simulink library "EoM_6DoF"  (R2021b)
settings: Solver=VariableStepAuto  StartTime=0.0  StopTime=10.0  RelTol=1e-3
undefined symbols (not defined in the file or in its folder): g, p0, phi0, psi0, q0, r0, theta0, u0, v0, w0, X0, Y0, Z0
libraries: EqMpro x12
settings Model: Creator=setup  LastModifiedBy=dmgp1

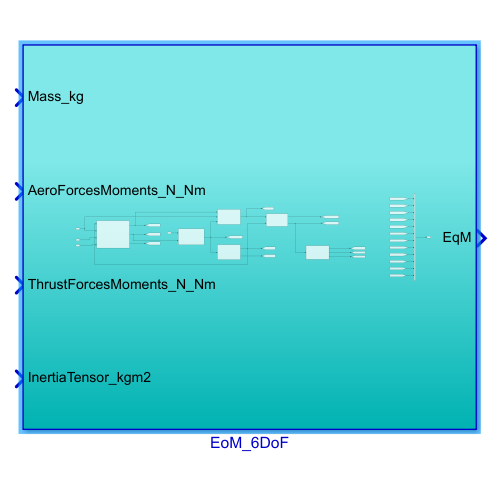
[thumbnail: Simulink's stored preview of the top-level diagram]
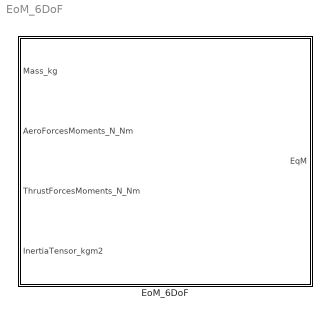
== system EoM_6DoF ==
  EoM_6DoF : Subsystem

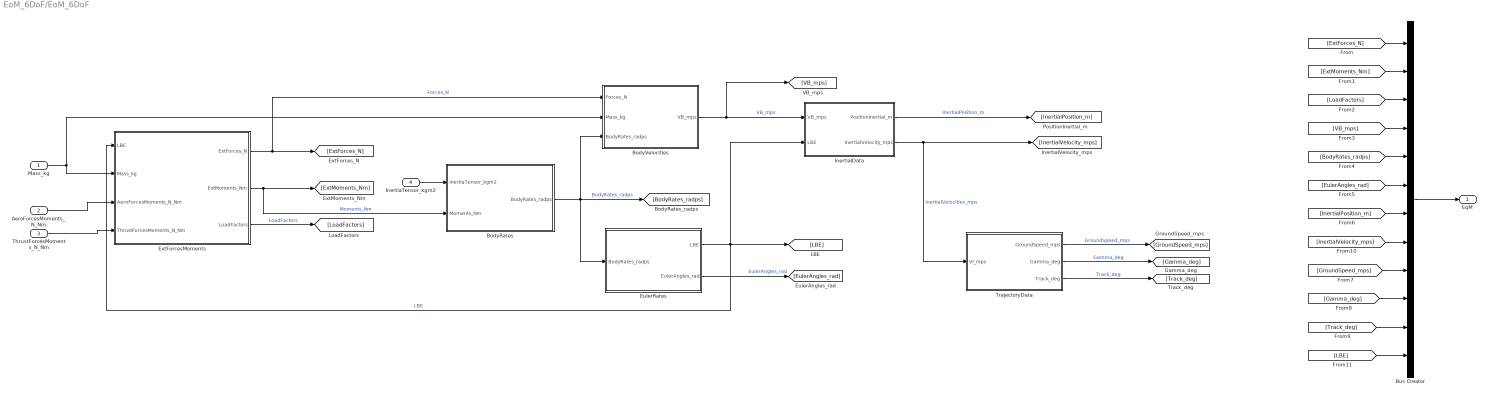
== system EoM_6DoF/EoM_6DoF ==
  Mass_kg : Inport  PortDimensions=[1]
  AeroForcesMoments_N_Nm : Inport  Port=2  PortDimensions=[6]
  ThrustForcesMoments_N_Nm : Inport  Port=3  PortDimensions=[6]
  InertiaTensor_kgm2 : Inport  Port=4
  BodyRates : Subsystem
  BodyVelocities : Subsystem
  Bus Creator : BusCreator  Inputs=12
  EulerRates : Subsystem
  ExtForcesMoments : Subsystem
  InertialData : Subsystem
  TrajectoryData : Subsystem
  EqM : Outport
  wires:
  ExtForcesMoments/3(LoadFactors) -> [LoadFactors]  "LoadFactors"
  BodyVelocities/1(VB_mps) -> [VB_mps], InertialData/1(VB_mps)  "VB_mps"
  [LBE] -> Bus Creator/12
  ThrustForcesMoments_N_Nm/1 -> ExtForcesMoments/4(ThrustForcesMoments_N_Nm)
  [Track_deg] -> Bus Creator/11
  Bus Creator/1 -> EqM/1
  TrajectoryData/3(Track_deg) -> [Track_deg]  "Track_deg"
  AeroForcesMoments_N_Nm/1 -> ExtForcesMoments/3(AeroForcesMoments_N_Nm)
  [ExtForces_N] -> Bus Creator/1
  ExtForcesMoments/1(ExtForces_N) -> BodyVelocities/1(Forces_N), [ExtForces_N]  "Forces_N"
  [Gamma_deg] -> Bus Creator/10
  [LoadFactors] -> Bus Creator/3
  [InertialPosition_m] -> Bus Creator/7
  [VB_mps] -> Bus Creator/4
  BodyRates/1(BodyRates_radps) -> [BodyRates_radps], EulerRates/1(BodyRates_radps), BodyVelocities/3(BodyRates_radps)  "BodyRates_radps"
  Mass_kg/1 -> ExtForcesMoments/2(Mass_kg), BodyVelocities/2(Mass_kg)
  EulerRates/1(LBE) -> ExtForcesMoments/1(LBE), [LBE], InertialData/2(LBE)  "LBE"
  InertialData/1(PositionInertial_m) -> [InertialPosition_m]  "InertialPosition_m"
  ExtForcesMoments/2(ExtMoments_Nm) -> BodyRates/2(Moments_Nm), [ExtMoments_Nm]  "Moments_Nm"
  [GroundSpeed_mps] -> Bus Creator/9
  EulerRates/2(EulerAngles_rad) -> [EulerAngles_rad]  "EulerAngles_rad"
  [InertialVelocity_mps] -> Bus Creator/8
  InertialData/2(InertialVelocity_mps) -> [InertialVelocity_mps], TrajectoryData/1(VI_mps)  "InertialVelocities_mps"
  [ExtMoments_Nm] -> Bus Creator/2
  TrajectoryData/2(Gamma_deg) -> [Gamma_deg]  "Gamma_deg"
  InertiaTensor_kgm2/1 -> BodyRates/1(InertiaTensor_kgm2)
  [EulerAngles_rad] -> Bus Creator/6
  [BodyRates_radps] -> Bus Creator/5
  TrajectoryData/1(GroundSpeed_mps) -> [GroundSpeed_mps]  "GroundSpeed_mps"

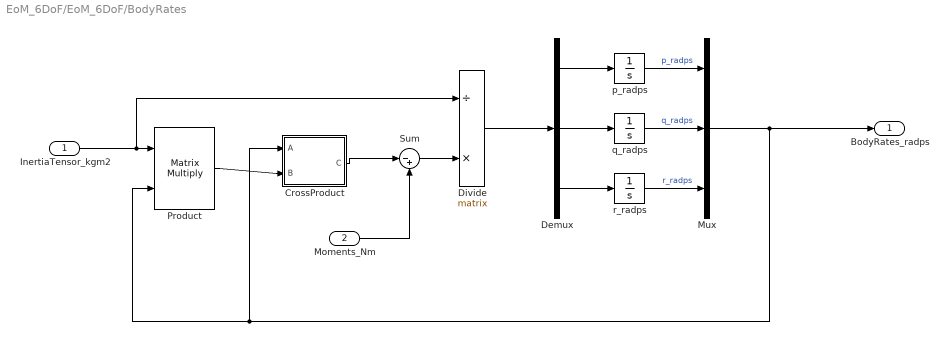
== system EoM_6DoF/EoM_6DoF/BodyRates ==
  InertiaTensor_kgm2 : Inport
  Moments_Nm : Inport  Port=2  PortDimensions=[3]
  CrossProduct : Subsystem
  Demux : Demux  Outputs=3
  Divide : Product  Inputs=/*  Multiplication=Matrix(*)
  Mux : Mux  Inputs=3
  Product : Product  Multiplication=Matrix(*)
  Sum : Sum  Inputs=|-+
  p_radps : Integrator  InitialCondition=p0  ContinuousStateAttributes='p_radps'
  q_radps : Integrator  InitialCondition=q0  ContinuousStateAttributes='q_radps'
  r_radps : Integrator  InitialCondition=r0  ContinuousStateAttributes='r_radps'
  BodyRates_radps : Outport  PortDimensions=[3]
  wires:
  Demux/3 -> r_radps/1
  InertiaTensor_kgm2/1 -> Divide/1, Product/1
  Mux/1 -> BodyRates_radps/1, Product/2, CrossProduct/1(A)
  Product/1 -> CrossProduct/2(B)
  Moments_Nm/1 -> Sum/2
  r_radps/1 -> Mux/3  "r_radps"
  CrossProduct/1(C) -> Sum/1
  Sum/1 -> Divide/2
  q_radps/1 -> Mux/2  "q_radps"
  Demux/1 -> p_radps/1
  p_radps/1 -> Mux/1  "p_radps"
  Demux/2 -> q_radps/1
  Divide/1 -> Demux/1

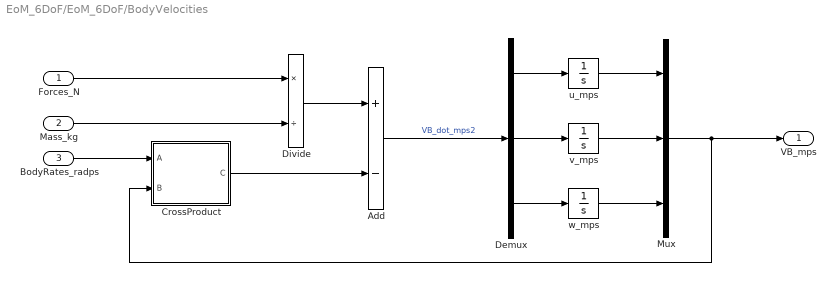
== system EoM_6DoF/EoM_6DoF/BodyVelocities ==
  Forces_N : Inport  PortDimensions=[3]
  Mass_kg : Inport  Port=2  PortDimensions=[1]
  BodyRates_radps : Inport  Port=3  PortDimensions=[3]
  Add : Sum  Inputs=+-
  CrossProduct : Subsystem
  Demux : Demux  Outputs=3
  Divide : Product  Inputs=*/
  Mux : Mux  Inputs=3
  u_mps : Integrator  InitialCondition=u0  ContinuousStateAttributes='u_mps'
  v_mps : Integrator  InitialCondition=v0  ContinuousStateAttributes='v_mps'
  w_mps : Integrator  InitialCondition=w0  ContinuousStateAttributes='w_mps'
  VB_mps : Outport  PortDimensions=[3]
  wires:
  Mux/1 -> VB_mps/1, CrossProduct/2(B)
  Forces_N/1 -> Divide/1
  u_mps/1 -> Mux/1
  Mass_kg/1 -> Divide/2
  Add/1 -> Demux/1  "VB_dot_mps2"
  Divide/1 -> Add/1
  w_mps/1 -> Mux/3
  Demux/1 -> u_mps/1
  CrossProduct/1(C) -> Add/2
  Demux/2 -> v_mps/1
  Demux/3 -> w_mps/1
  v_mps/1 -> Mux/2
  BodyRates_radps/1 -> CrossProduct/1(A)

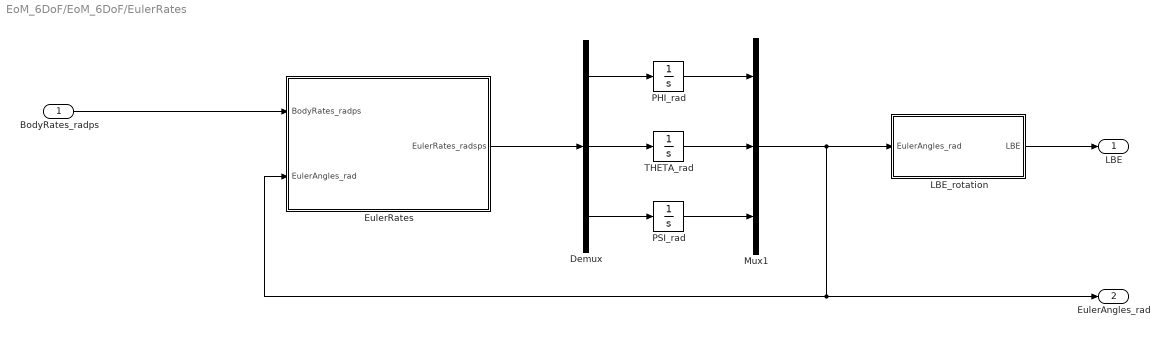
== system EoM_6DoF/EoM_6DoF/EulerRates ==
  BodyRates_radps : Inport  PortDimensions=[3]
  Demux : Demux  Outputs=3
  EulerRates : Subsystem
  LBE_rotation : Subsystem
  Mux1 : Mux  Inputs=3
  PHI_rad : Integrator  InitialCondition=phi0  ContinuousStateAttributes='PHI_rad'
  PSI_rad : Integrator  InitialCondition=psi0  ContinuousStateAttributes='PSI_rad'
  THETA_rad : Integrator  InitialCondition=theta0  ContinuousStateAttributes='THETA_rad'
  LBE : Outport
  EulerAngles_rad : Outport  Port=2
  wires:
  Mux1/1 -> EulerAngles_rad/1, EulerRates/2(EulerAngles_rad), LBE_rotation/1(EulerAngles_rad)
  LBE_rotation/1(LBE) -> LBE/1
  PHI_rad/1 -> Mux1/1
  EulerRates/1(EulerRates_radsps) -> Demux/1
  THETA_rad/1 -> Mux1/2
  PSI_rad/1 -> Mux1/3
  Demux/2 -> THETA_rad/1
  Demux/3 -> PSI_rad/1
  Demux/1 -> PHI_rad/1
  BodyRates_radps/1 -> EulerRates/1(BodyRates_radps)

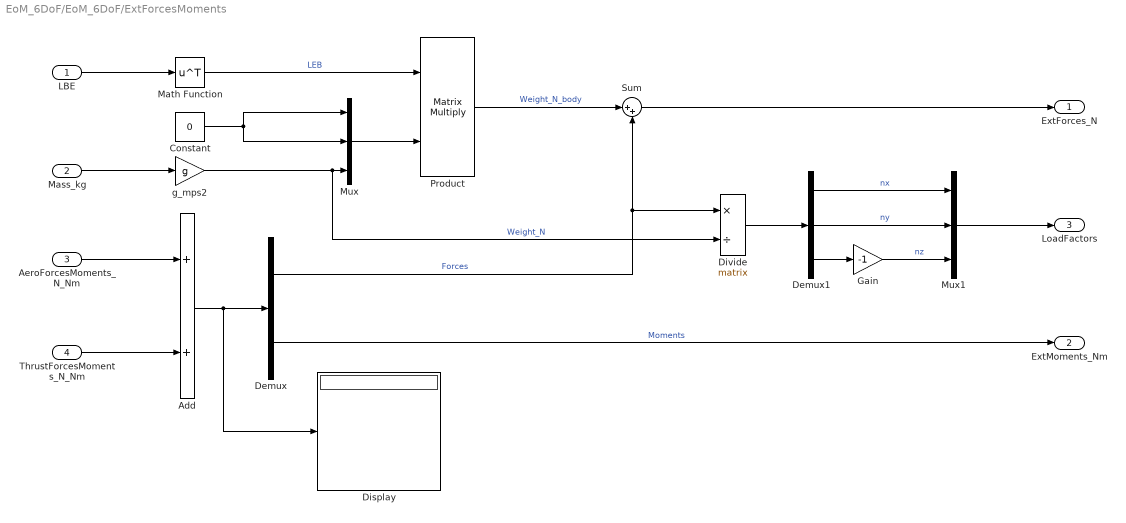
== system EoM_6DoF/EoM_6DoF/ExtForcesMoments ==
  LBE : Inport
  Mass_kg : Inport  Port=2  PortDimensions=[1]
  AeroForcesMoments_N_Nm : Inport  Port=3  PortDimensions=[6]
  ThrustForcesMoments_N_Nm : Inport  Port=4  PortDimensions=[6]
  Add : Sum
  Constant : Constant  Value=0
  Demux : Demux  Outputs=2
  Demux1 : Demux  Outputs=3
  Display : Display
  Divide : Product  Inputs=*/  Multiplication=Matrix(*)
  Gain : Gain  Gain=-1
  Math Function : Math  Operator=transpose  SignedPower=on  SaturateOnIntegerOverflow=on
  Mux : Mux  Inputs=3
  Mux1 : Mux  Inputs=3
  Product : Product  Multiplication=Matrix(*)
  Sum : Sum  Inputs=|++
  g_mps2 : Gain  Gain=g
  ExtForces_N : Outport  PortDimensions=[3]
  ExtMoments_Nm : Outport  Port=2  PortDimensions=[3]
  LoadFactors : Outport  Port=3  PortDimensions=[3]
  wires:
  Demux/2 -> ExtMoments_Nm/1  "Moments"
  AeroForcesMoments_N_Nm/1 -> Add/1
  Divide/1 -> Demux1/1
  Demux/1 -> Sum/2, Divide/1  "Forces"
  Sum/1 -> ExtForces_N/1
  Mux1/1 -> LoadFactors/1
  ThrustForcesMoments_N_Nm/1 -> Add/2
  Constant/1 -> Mux/1, Mux/2
  Add/1 -> Display/1, Demux/1
  Math Function/1 -> Product/1  "LEB"
  Mass_kg/1 -> g_mps2/1
  Mux/1 -> Product/2
  g_mps2/1 -> Mux/3, Divide/2  "Weight_N"
  Demux1/3 -> Gain/1
  Product/1 -> Sum/1  "Weight_N_body"
  Demux1/1 -> Mux1/1  "nx"
  Gain/1 -> Mux1/3  "nz"
  LBE/1 -> Math Function/1
  Demux1/2 -> Mux1/2  "ny"

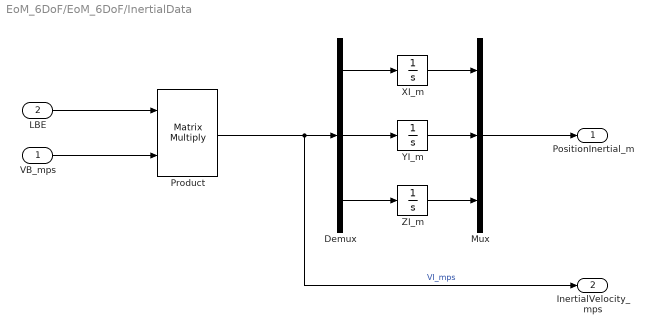
== system EoM_6DoF/EoM_6DoF/InertialData ==
  VB_mps : Inport
  LBE : Inport  Port=2
  Demux : Demux  Outputs=3
  Mux : Mux  Inputs=3
  Product : Product  Multiplication=Matrix(*)
  XI_m : Integrator  InitialCondition=X0  ContinuousStateAttributes='XI_m'
  YI_m : Integrator  InitialCondition=Y0  ContinuousStateAttributes='YI_m'
  ZI_m : Integrator  InitialCondition=Z0  ContinuousStateAttributes='ZI_m'
  PositionInertial_m : Outport
  InertialVelocity_mps : Outport  Port=2
  wires:
  VB_mps/1 -> Product/2
  Mux/1 -> PositionInertial_m/1
  XI_m/1 -> Mux/1
  Demux/1 -> XI_m/1
  Product/1 -> InertialVelocity_mps/1, Demux/1  "VI_mps"
  LBE/1 -> Product/1
  ZI_m/1 -> Mux/3
  Demux/3 -> ZI_m/1
  YI_m/1 -> Mux/2
  Demux/2 -> YI_m/1

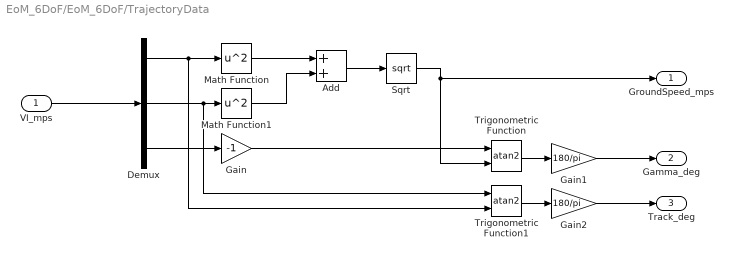
== system EoM_6DoF/EoM_6DoF/TrajectoryData ==
  VI_mps : Inport
  Add : Sum
  Demux : Demux  Outputs=3
  Gain : Gain  Gain=-1
  Gain1 : Gain  Gain=180/pi
  Gain2 : Gain  Gain=180/pi
  Math Function : Math  Operator=square  SignedPower=on  SaturateOnIntegerOverflow=on
  Math Function1 : Math  Operator=square  SignedPower=on  SaturateOnIntegerOverflow=on
  Sqrt : Sqrt  SaturateOnIntegerOverflow=on
  Trigonometric Function : Trigonometry  Operator=atan2
  Trigonometric Function1 : Trigonometry  Operator=atan2
  GroundSpeed_mps : Outport
  Gamma_deg : Outport  Port=2
  Track_deg : Outport  Port=3
  wires:
  Gain2/1 -> Track_deg/1
  Trigonometric Function/1 -> Gain1/1
  Gain1/1 -> Gamma_deg/1
  VI_mps/1 -> Demux/1
  Sqrt/1 -> GroundSpeed_mps/1, Trigonometric Function/2
  Math Function1/1 -> Add/2
  Demux/2 -> Math Function1/1, Trigonometric Function1/1
  Add/1 -> Sqrt/1
  Math Function/1 -> Add/1
  Demux/3 -> Gain/1
  Demux/1 -> Math Function/1, Trigonometric Function1/2
  Gain/1 -> Trigonometric Function/1
  Trigonometric Function1/1 -> Gain2/1

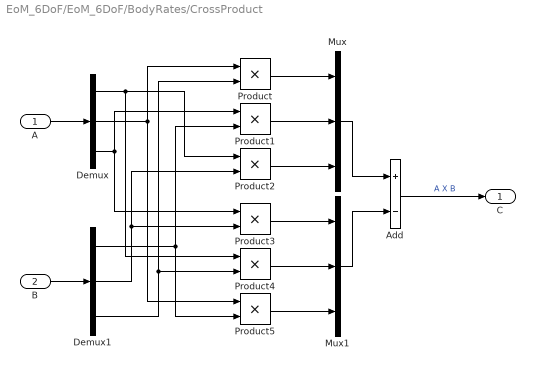
== system EoM_6DoF/EoM_6DoF/BodyRates/CrossProduct ==
  A : Inport
  B : Inport  Port=2
  Add : Sum  Inputs=+-
  Demux : Demux  Outputs=3
  Demux1 : Demux  Outputs=3
  Mux : Mux  Inputs=3
  Mux1 : Mux  Inputs=3
  Product{,1..5} (6 alike) : Product
  C : Outport
  wires:
  Demux/2 -> Product/1, Product5/1
  Demux1/2 -> Product2/2, Product3/2
  Product3/1 -> Mux1/1
  Demux/1 -> Product2/1, Product4/1
  Product4/1 -> Mux1/2
  Product/1 -> Mux/1
  Product5/1 -> Mux1/3
  Demux/3 -> Product1/1, Product3/1
  Product2/1 -> Mux/3
  Product1/1 -> Mux/2
  A/1 -> Demux/1
  Mux1/1 -> Add/2
  Demux1/1 -> Product1/2, Product5/2
  Demux1/3 -> Product/2, Product4/2
  B/1 -> Demux1/1
  Mux/1 -> Add/1
  Add/1 -> C/1  "A X B"

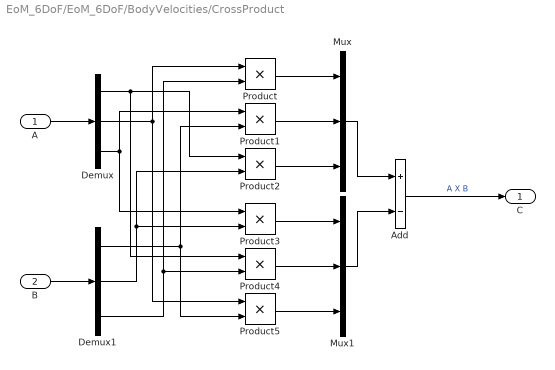
== system EoM_6DoF/EoM_6DoF/BodyVelocities/CrossProduct ==
  A : Inport
  B : Inport  Port=2
  Add : Sum  Inputs=+-
  Demux : Demux  Outputs=3
  Demux1 : Demux  Outputs=3
  Mux : Mux  Inputs=3
  Mux1 : Mux  Inputs=3
  Product{,1..5} (6 alike) : Product
  C : Outport
  wires:
  A/1 -> Demux/1
  Mux/1 -> Add/1
  Demux/3 -> Product1/1, Product3/1
  Product5/1 -> Mux1/3
  Demux1/2 -> Product2/2, Product3/2
  Demux1/3 -> Product/2, Product4/2
  Product4/1 -> Mux1/2
  Demux1/1 -> Product1/2, Product5/2
  Demux/1 -> Product2/1, Product4/1
  B/1 -> Demux1/1
  Add/1 -> C/1  "A X B"
  Demux/2 -> Product/1, Product5/1
  Product/1 -> Mux/1
  Product1/1 -> Mux/2
  Product2/1 -> Mux/3
  Mux1/1 -> Add/2
  Product3/1 -> Mux1/1

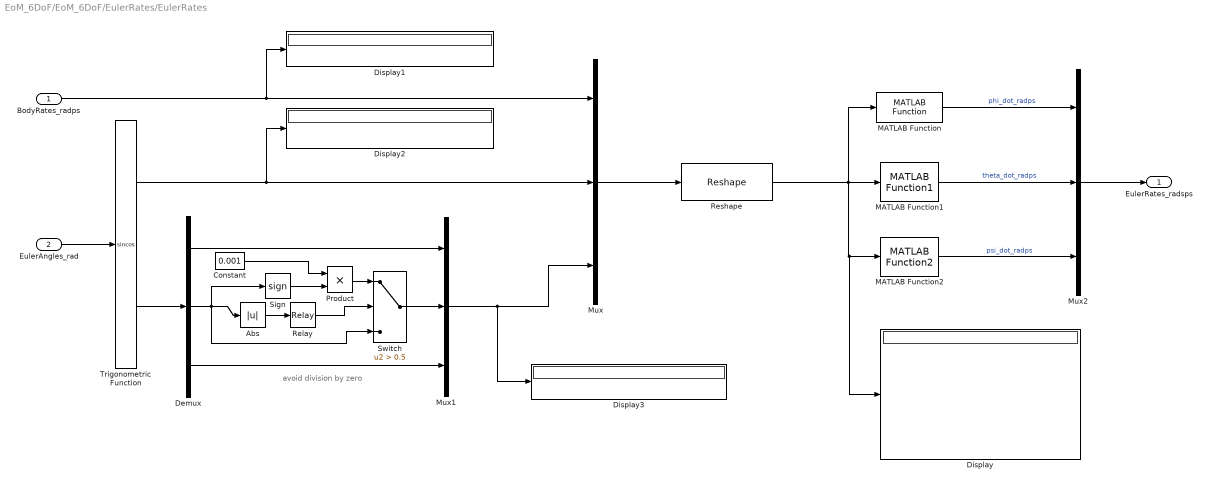
== system EoM_6DoF/EoM_6DoF/EulerRates/EulerRates ==
  note: avoid division by zero
  BodyRates_radps : Inport  PortDimensions=[3]
  EulerAngles_rad : Inport  Port=2  PortDimensions=[3]
  Abs : Abs
  Constant : Constant  Value=0.001
  Demux : Demux  Outputs=3
  Display{,1..3} (4 alike) : Display
  MATLAB Function : EqMpro/EqM/EulerAngles/EulerRates/MATLAB Function  SystemSampleTime=-1  VariantActivationTime=update diagram  Latency=0  AutoFrameSizeCalculation=off
  MATLAB Function1 : EqMpro/EqM/EulerAngles/EulerRates/MATLAB Function1  SystemSampleTime=-1  VariantActivationTime=update diagram  Latency=0  AutoFrameSizeCalculation=off
  MATLAB Function2 : EqMpro/EqM/EulerAngles/EulerRates/MATLAB Function2  SystemSampleTime=-1  VariantActivationTime=update diagram  Latency=0  AutoFrameSizeCalculation=off
  Mux : Mux  Inputs=3
  Mux1 : Mux  Inputs=3
  Mux2 : Mux  Inputs=3
  Product : Product
  Relay : Relay  OnSwitchValue=.001  OffSwitchValue=0  OnOutputValue=0  OffOutputValue=1
  Reshape : Reshape
  Sign : Signum
  Switch : Switch  Criteria=u2 > Threshold  Threshold=0.5
  Trigonometric Function : Trigonometry  Operator=sincos
  EulerRates_radsps : Outport  PortDimensions=[3]
  wires:
  Abs/1 -> Relay/1
  EulerAngles_rad/1 -> Trigonometric Function/1
  Demux/2 -> Switch/3, Abs/1, Sign/1
  Relay/1 -> Switch/2
  Switch/1 -> Mux1/2
  Sign/1 -> Product/2
  Demux/3 -> Mux1/3
  MATLAB Function2/1 -> Mux2/3  "psi_dot_radps"
  MATLAB Function1/1 -> Mux2/2  "theta_dot_radps"
  BodyRates_radps/1 -> Mux/1, Display1/1
  Trigonometric Function/2 -> Demux/1
  MATLAB Function/1 -> Mux2/1  "phi_dot_radps"
  Product/1 -> Switch/1
  Mux2/1 -> EulerRates_radsps/1
  Trigonometric Function/1 -> Mux/2, Display2/1
  Constant/1 -> Product/1
  Mux1/1 -> Display3/1, Mux/3
  Demux/1 -> Mux1/1
  Mux/1 -> Reshape/1
  Reshape/1 -> Display/1, MATLAB Function2/1, MATLAB Function/1, MATLAB Function1/1

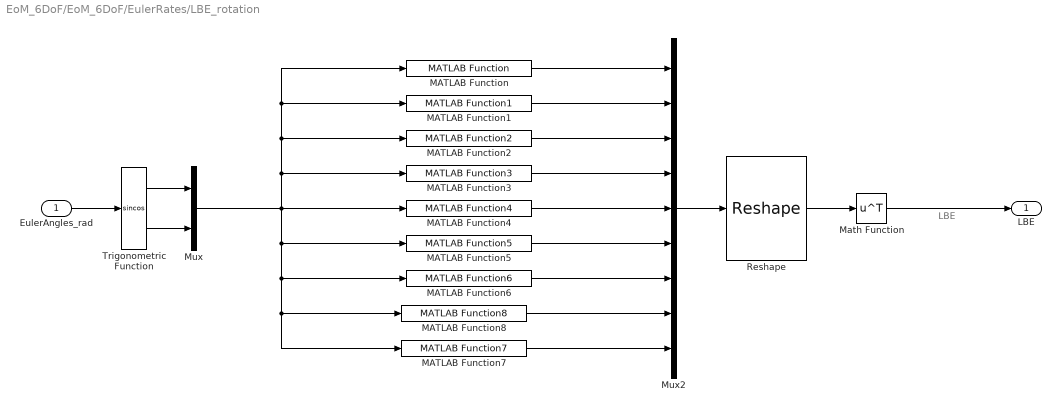
== system EoM_6DoF/EoM_6DoF/EulerRates/LBE_rotation ==
  note: LBE
  EulerAngles_rad : Inport
  MATLAB Function : EqMpro/EqM/EulerAngles/LBE_rotation/MATLAB Function  SystemSampleTime=-1  VariantActivationTime=update diagram  Latency=0  AutoFrameSizeCalculation=off
  MATLAB Function1 : EqMpro/EqM/EulerAngles/LBE_rotation/MATLAB Function1  SystemSampleTime=-1  VariantActivationTime=update diagram  Latency=0  AutoFrameSizeCalculation=off
  MATLAB Function2 : EqMpro/EqM/EulerAngles/LBE_rotation/MATLAB Function2  SystemSampleTime=-1  VariantActivationTime=update diagram  Latency=0  AutoFrameSizeCalculation=off
  MATLAB Function3 : EqMpro/EqM/EulerAngles/LBE_rotation/MATLAB Function3  SystemSampleTime=-1  VariantActivationTime=update diagram  Latency=0  AutoFrameSizeCalculation=off
  MATLAB Function4 : EqMpro/EqM/EulerAngles/LBE_rotation/MATLAB Function4  SystemSampleTime=-1  VariantActivationTime=update diagram  Latency=0  AutoFrameSizeCalculation=off
  MATLAB Function5 : EqMpro/EqM/EulerAngles/LBE_rotation/MATLAB Function5  SystemSampleTime=-1  VariantActivationTime=update diagram  Latency=0  AutoFrameSizeCalculation=off
  MATLAB Function6 : EqMpro/EqM/EulerAngles/LBE_rotation/MATLAB Function6  SystemSampleTime=-1  VariantActivationTime=update diagram  Latency=0  AutoFrameSizeCalculation=off
  MATLAB Function7 : EqMpro/EqM/EulerAngles/LBE_rotation/MATLAB Function7  SystemSampleTime=-1  VariantActivationTime=update diagram  Latency=0  AutoFrameSizeCalculation=off
  MATLAB Function8 : EqMpro/EqM/EulerAngles/LBE_rotation/MATLAB Function8  SystemSampleTime=-1  VariantActivationTime=update diagram  Latency=0  AutoFrameSizeCalculation=off
  Math Function : Math  Operator=transpose  SignedPower=on  SaturateOnIntegerOverflow=on
  Mux : Mux  Inputs=2
  Mux2 : Mux  Inputs=9
  Reshape : Reshape  OutputDimensionality=Customize  OutputDimensions=[3,3]
  Trigonometric Function : Trigonometry  Operator=sincos
  LBE : Outport
  wires:
  Math Function/1 -> LBE/1
  Mux/1 -> MATLAB Function3/1, MATLAB Function2/1, MATLAB Function1/1, MATLAB Function/1, MATLAB Function4/1, MATLAB Function5/1, MATLAB Function6/1, MATLAB Function7/1, MATLAB Function8/1
  Mux2/1 -> Reshape/1
  MATLAB Function3/1 -> Mux2/4
  MATLAB Function6/1 -> Mux2/7
  MATLAB Function8/1 -> Mux2/8
  Reshape/1 -> Math Function/1
  MATLAB Function2/1 -> Mux2/3
  EulerAngles_rad/1 -> Trigonometric Function/1
  Trigonometric Function/1 -> Mux/1
  MATLAB Function7/1 -> Mux2/9
  MATLAB Function1/1 -> Mux2/2
  MATLAB Function5/1 -> Mux2/6
  Trigonometric Function/2 -> Mux/2
  MATLAB Function/1 -> Mux2/1
  MATLAB Function4/1 -> Mux2/5
